simulink subsystem "esc_status_format"  (R2024a)
settings: Solver=VariableStepAuto  StartTime=0.0  StopTime=10.0  RelTol=1e-3
settings Model: Creator=gurt1  LastModifiedBy=gurt1

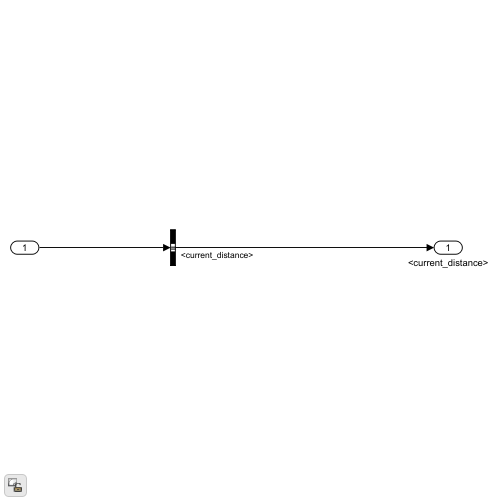
[thumbnail: Simulink's stored preview of the top-level diagram]
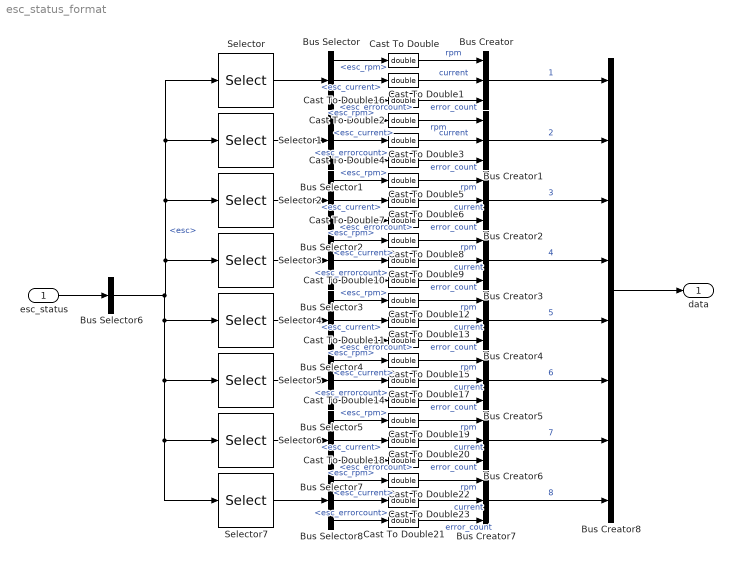
== system esc_status_format ==
  esc_status : Inport
  Bus Creator{,1..7} (8 alike) : BusCreator  Inputs=3
  Bus Creator8 : BusCreator  Inputs=8
  Bus Selector{,1..5,7..8} (8 alike) : BusSelector  OutputSignals=esc_rpm,esc_current,esc_errorcount
  Bus Selector6 : BusSelector  OutputSignals=esc
  Cast To Double{,1..23} (24 alike) : DataTypeConversion  OutDataTypeStr=double  SaturateOnIntegerOverflow=off  RndMeth=Floor
  Selector : Selector  InputPortWidth=8  IndexOptions=Index vector (dialog)  Indices=[1]  OutputSizes=1
  Selector1 : Selector  InputPortWidth=8  IndexOptions=Index vector (dialog)  Indices=[2]  OutputSizes=1
  Selector2 : Selector  InputPortWidth=8  IndexOptions=Index vector (dialog)  Indices=[3]  OutputSizes=1
  Selector3 : Selector  InputPortWidth=8  IndexOptions=Index vector (dialog)  Indices=[4]  OutputSizes=1
  Selector4 : Selector  InputPortWidth=8  IndexOptions=Index vector (dialog)  Indices=[5]  OutputSizes=1
  Selector5 : Selector  InputPortWidth=8  IndexOptions=Index vector (dialog)  Indices=[6]  OutputSizes=1
  Selector6 : Selector  InputPortWidth=8  IndexOptions=Index vector (dialog)  Indices=[7]  OutputSizes=1
  Selector7 : Selector  InputPortWidth=8  IndexOptions=Index vector (dialog)  Indices=[8]  OutputSizes=1
  data : Outport
  wires:
  Bus Selector6/1 -> Selector/1, Selector1/1, Selector2/1, Selector3/1, Selector4/1, Selector5/1, Selector6/1, Selector7/1  "<esc>"
  esc_status/1 -> Bus Selector6/1
  Selector/1 -> Bus Selector/1
  Selector1/1 -> Bus Selector1/1
  Selector3/1 -> Bus Selector3/1
  Selector2/1 -> Bus Selector2/1
  Selector4/1 -> Bus Selector4/1
  Selector5/1 -> Bus Selector5/1
  Selector7/1 -> Bus Selector8/1
  Selector6/1 -> Bus Selector7/1
  Bus Selector/1 -> Cast To Double/1  "<esc_rpm>"
  Bus Selector/2 -> Cast To Double1/1  "<esc_current>"
  Cast To Double/1 -> Bus Creator/1  "rpm"
  Cast To Double1/1 -> Bus Creator/2  "current"
  Bus Creator/1 -> Bus Creator8/1  "1"
  Bus Creator1/1 -> Bus Creator8/2  "2"
  Bus Creator2/1 -> Bus Creator8/3  "3"
  Bus Creator3/1 -> Bus Creator8/4  "4"
  Bus Creator4/1 -> Bus Creator8/5  "5"
  Bus Creator5/1 -> Bus Creator8/6  "6"
  Bus Creator6/1 -> Bus Creator8/7  "7"
  Bus Creator8/1 -> data/1
  Bus Selector/3 -> Cast To Double16/1  "<esc_errorcount>"
  Cast To Double16/1 -> Bus Creator/3  "error_count"
  Cast To Double4/1 -> Bus Creator1/3  "error_count"
  Bus Selector1/3 -> Cast To Double4/1  "<esc_errorcount>"
  Cast To Double3/1 -> Bus Creator1/2  "current"
  Cast To Double2/1 -> Bus Creator1/1  "rpm"
  Bus Selector1/2 -> Cast To Double3/1  "<esc_current>"
  Bus Selector1/1 -> Cast To Double2/1  "<esc_rpm>"
  Bus Selector2/1 -> Cast To Double5/1  "<esc_rpm>"
  Bus Selector2/2 -> Cast To Double6/1  "<esc_current>"
  Cast To Double5/1 -> Bus Creator2/1  "rpm"
  Cast To Double6/1 -> Bus Creator2/2  "current"
  Bus Selector2/3 -> Cast To Double7/1  "<esc_errorcount>"
  Cast To Double7/1 -> Bus Creator2/3  "error_count"
  Cast To Double10/1 -> Bus Creator3/3  "error_count"
  Bus Selector3/3 -> Cast To Double10/1  "<esc_errorcount>"
  Cast To Double9/1 -> Bus Creator3/2  "current"
  Cast To Double8/1 -> Bus Creator3/1  "rpm"
  Bus Selector3/2 -> Cast To Double9/1  "<esc_current>"
  Bus Selector3/1 -> Cast To Double8/1  "<esc_rpm>"
  Bus Selector4/1 -> Cast To Double12/1  "<esc_rpm>"
  Bus Selector4/2 -> Cast To Double13/1  "<esc_current>"
  Cast To Double12/1 -> Bus Creator4/1  "rpm"
  Cast To Double13/1 -> Bus Creator4/2  "current"
  Bus Selector4/3 -> Cast To Double11/1  "<esc_errorcount>"
  Cast To Double11/1 -> Bus Creator4/3  "error_count"
  Cast To Double14/1 -> Bus Creator5/3  "error_count"
  Bus Selector5/3 -> Cast To Double14/1  "<esc_errorcount>"
  Cast To Double17/1 -> Bus Creator5/2  "current"
  Cast To Double15/1 -> Bus Creator5/1  "rpm"
  Bus Selector5/2 -> Cast To Double17/1  "<esc_current>"
  Bus Selector5/1 -> Cast To Double15/1  "<esc_rpm>"
  Bus Selector7/1 -> Cast To Double19/1  "<esc_rpm>"
  Bus Selector7/2 -> Cast To Double20/1  "<esc_current>"
  Cast To Double19/1 -> Bus Creator6/1  "rpm"
  Cast To Double20/1 -> Bus Creator6/2  "current"
  Bus Selector7/3 -> Cast To Double18/1  "<esc_errorcount>"
  Cast To Double18/1 -> Bus Creator6/3  "error_count"
  Cast To Double21/1 -> Bus Creator7/3  "error_count"
  Bus Selector8/3 -> Cast To Double21/1  "<esc_errorcount>"
  Cast To Double23/1 -> Bus Creator7/2  "current"
  Cast To Double22/1 -> Bus Creator7/1  "rpm"
  Bus Selector8/2 -> Cast To Double23/1  "<esc_current>"
  Bus Selector8/1 -> Cast To Double22/1  "<esc_rpm>"
  Bus Creator7/1 -> Bus Creator8/8  "8"
